simulink model "quadcopter_package_delivery"  (R2025a)
settings: Solver=ode23t  StartTime=0.0  StopTime=timespot_spl(end)+2  FixedStep=0.01  MaxStep=1e-2  RelTol=1e-3  AbsTol=1e-3
model workspace (MATLAB code in the model file):
  | load('xy_data_membrane.mat');
values from neighbouring files (symbols this model uses):
  air_rho = 1.225    [quadcopter_package_parameters.m]
  battery_capacity = 7.6*3    (= 22.8)    [quadcopter_package_parameters.m]
  filtD_altitude = 10000    [quadcopter_package_parameters.m]
  filtD_attitude = 1000    [quadcopter_package_parameters.m]
  filtD_motor = 10000    [quadcopter_package_parameters.m]
  filtD_yaw = 100    [quadcopter_package_parameters.m]
  filtM_altitude = 0.05    [quadcopter_package_parameters.m]
  filtM_attitude = 0.01    [quadcopter_package_parameters.m]
  filtM_yaw = 0.01    [quadcopter_package_parameters.m]
  filtSpd_motor = 0.001    [quadcopter_package_parameters.m]
  kd_altitude = 0.35    [quadcopter_package_parameters.m]
  kd_attitude = 78.2000*2    (= 156.4)    [quadcopter_package_parameters.m]
  kd_motor = 0    [quadcopter_package_parameters.m]
  kd_yaw = 78.2000*0.01    (= 0.782)    [quadcopter_package_parameters.m]
  ki_altitude = 0.07    [quadcopter_package_parameters.m]
  ki_attitude = 5.9203    [quadcopter_package_parameters.m]
  ki_motor = 4.50000e-4    (= 0.00045)    [quadcopter_package_parameters.m]
  ki_yaw = 5.9203*0.01    (= 0.059203)    [quadcopter_package_parameters.m]
  kp_altitude = 0.27    [quadcopter_package_parameters.m]
  kp_attitude = 128.505    [quadcopter_package_parameters.m]
  kp_motor = 0.00375    [quadcopter_package_parameters.m]
  kp_yaw = 25.7010*4*2    (= 205.608)    [quadcopter_package_parameters.m]
  limit_altitude = 10    [quadcopter_package_parameters.m]
  limit_attitude = 800    [quadcopter_package_parameters.m]
  limit_motor = 0.25    [quadcopter_package_parameters.m]
  limit_yaw = 20    [quadcopter_package_parameters.m]
  N = size(targetsENU,1)    [ARCsim.m]    (also in build_uav_virtcam_sim.m = size(worldPts,1))
  pkgDensity = 1/(pkgSize(1)*pkgSize(2)*pkgSize(3))    [quadcopter_package_parameters.m]
  pkgSize = [1 1 1]*0.14    [quadcopter_package_parameters.m]
  planedepth = 0.2    [quadcopter_package_parameters.m]
  s = dbstack('-completenames')    [build_uav_virtcam_sim.m]
  wind_speed = 0    [quadcopter_package_parameters.m]
  X = center(1) + r*cos(th)    [build_uav_virtcam_sim.m]
  Y = center(2) + r*sin(th)    [build_uav_virtcam_sim.m]
  Z = center(3) + z - hgt/2    [build_uav_virtcam_sim.m]
undefined symbols (not defined in the file or in its folder): drone_leg, propeller, qc_motor, qd_area, qd_drag, waypoints
libraries: sm_lib x77, nesl_utility x30, fl_lib x13, slpidlib x11, quadcopter_library x6, ee_lib x4, simulink x2, batteryecm_lib x1
(part 5 of 5)

== system quadcopter_package_delivery/Quadcopter/Wind and Drag/Aerodynamic Drag/drag moment yaw ==
  v : Inport
  Constant : Constant  Value=rho_air/2
  Constant1 : Constant  Value=area_values.Yaw
  Constant2 : Constant  Value=drag_coeff.Yaw
  Gain : Gain  Gain=-1
  Product : Product  Inputs=5
  Sign : Signum  ZeroCross=off
  Square : Math  Operator=square
  f : Outport
  wires:
  Constant1/1 -> Product/2
  Sign/1 -> Product/5
  Constant/1 -> Product/1
  v/1 -> Sign/1, Square/1
  Gain/1 -> f/1
  Constant2/1 -> Product/3
  Square/1 -> Product/4
  Product/1 -> Gain/1

== matlab function quadcopter_package_delivery/Maneuver Controller/ErrorCalc ==
  data: dronePos input; ex output; objectPos input; ey output; ez output
function [ex,ey,ez] = ErrorCalc(dronePos, objectPos)
% dronePos: [x,y,z] from sensors (in inertial frame)
% objectPos: [x,y,z] target object position (in inertial frame)

% Compute position errors
ex = objectPos(1) - dronePos(1); % X error
ey = objectPos(2) - dronePos(2); % Y error
ez = objectPos(3) - dronePos(3); % Z error
end
